simulink model "tia1_controller"  (R2023b)
settings: Solver=VariableStepAuto  StartTime=0  StopTime=20e-4  RelTol=1e-3
values from neighbouring files (symbols this model uses):
  fNoiseSampling = 1 / (rpFloor(2,1) - rpFloor(1,1))    [Laser_n_PID_initializer.m]
  fsampling = 125e6    (= 125000000)    [Laser_n_PID_initializer.m]
  initialWaitTime = 8e-4    (= 0.0008)    [Laser_n_PID_initializer.m]
  nDelay = ceil(350*.5)    [Laser_n_PID_initializer.m]    (also in bode_check_stability_w_time_delay.m = 319)
  s = estimate_iir_transfer_function(x,y,3,1)    [linearModelization.m]
libraries: slctrl_linear x4, spsFirstOrderFilterLib x3, slpidlib x1
settings Model: Creator=lastline  LastModifiedBy=lastline

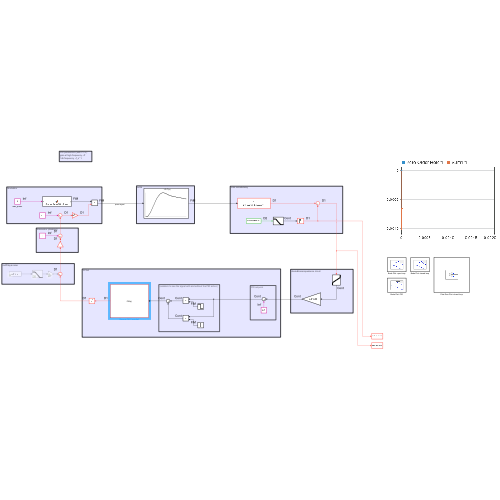
[thumbnail: Simulink's stored preview of the top-level diagram]
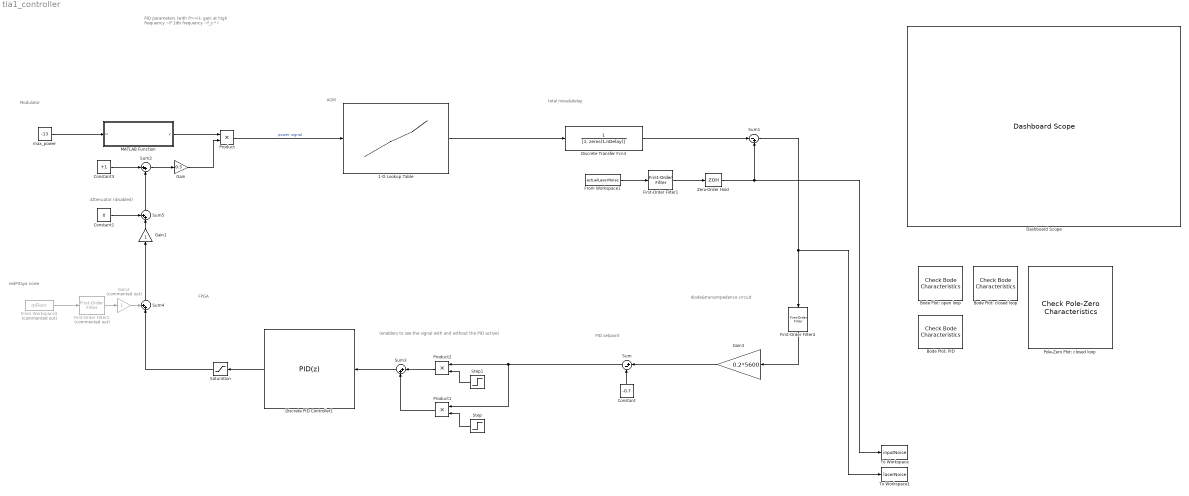
== system tia1_controller ==
  note: PID parameters (with P>>I):
      | gain at high frequency ~P
      | 1db frequency ~f_s * I
  note: PID setpoint
  note: (enablers to see the signal with and without the PID active)
  note: FPGA
  note: diode&transimpedance circuit
  note: Attenuator (disabled)
  note: AOM
  note: Modulator
  note: total noise&delay
  note: redPitaya noise
  1-D Lookup Table : Lookup_n-D  NumberOfTableDimensions=1  BreakpointsForDimension1=linspace(0, 1.58e-4, 250)  Table=0.7/0.0165796/(5600*0.2)*[0.00094876, 0.00102912, 0.00104173, 0.00106448, 0.00103857, 0.00100141, 0.00101933, 0.00100616, 0.00097746, 0.00121732, 0.00134761, 0.00150802, 0.00188835, 0.0021115 , 0.00246877, 0.00279502, 0.00315454, 0.0035255 , 0.00394097, 0.00436382, 0.00480437, 0.00527323, 0.00575644, 0.00627402, 0.00681823, 0.00736118, 0.00793556, 0.00852683, 0.00913098, 0.00972158, 0.01035586, 0.01102776, 0.0116796 , 0.01234212, 0.01306885, 0.0137567 , 0.01445381, 0.0151505 , 0.01585035, 0.01657956, 0.01728462, 0.01802811, 0.01875558, 0.01950813, 0.02025514, 0.02102895, 0.02180866, 0.02259664, 0.0233524 , 0.02406897, 0.02477072, 0.02553684, 0.02631157, 0.02703981, 0.02778477, 0.02851065, 0.02925919, 0.02997621, 0.03066793, 0.03135128, 0.0320296 , 0.03274458, 0.03341281, 0.03413072, 0.03476723, 0.0354006 , 0.03607709, 0.03668184, 0.03729911, 0.0378791 , 0.03846521, 0.0390453 , 0.03960121, 0.04011368, 0.04065807, 0.04118766, 0.04169539, 0.04217082, 0.0426283 , 0.04311696, 0.0435708 , 0.0439849 , 0.04437042, 0.04474889, 0.04514842, 0.04550796, 0.04586307, 0.04611688, 0.04647122, 0.04671718, 0.04707288, 0.04724069, 0.04745658, 0.04780167, 0.0479343 , 0.04808488, 0.04829364, 0.04849163, 0.04860279, 0.04865673, 0.04874706, 0.04886116, 0.04897224, 0.04908539, 0.04914333, 0.04916859, 0.04918415, 0.04919929, 0.04919949, 0.04918844, 0.0491581 , 0.04909332, 0.04902933, 0.04893137, 0.04879004, 0.04870624, 0.04865411, 0.04858254, 0.04848512, 0.04832172, 0.04815615, 0.04800017, 0.04790875, 0.04778889, 0.04761694, 0.04742341, 0.04726704, 0.04718501, 0.04700808, 0.04677664, 0.04662498, 0.04650092, 0.04634307, 0.04607253, 0.04590273, 0.04581645, 0.04568616, 0.04540447, 0.04523153, 0.0451333 , 0.04501928, 0.04482289, 0.04460957, 0.0444905 , 0.0444136 , 0.04426863, 0.04405665, 0.0439024 , 0.04381264, 0.04372158, 0.0436426 , 0.04347625, 0.04336099, 0.04321188, 0.04310523, 0.04304013, 0.04297429, 0.04289107, 0.04273544, 0.04258686, 0.0424759 , 0.04239794, 0.04236981, 0.04229522, 0.04221052, 0.04209073, 0.04197017, 0.04189005, 0.04178447, 0.04168274, 0.04166642, 0.04162506, 0.04155631, 0.04144807, 0.04133527, 0.04127493, 0.04118388, 0.04109912, 0.04101747, 0.04099294, 0.04096444, 0.04093825, 0.04089439, 0.04081889, 0.04076137, 0.04072337, 0.04064599, 0.0405364 , 0.04043972, 0.04039083, 0.04034431, 0.04030449, 0.04026617, 0.04022117, 0.04017923, 0.04012702, 0.04004417, 0.03997472, 0.03988416, 0.03978438, 0.03975578, 0.03968915, 0.03963203, 0.03959104, 0.03955679, 0.03953011, 0.03948652, 0.0394475 , 0.0393199 , 0.03924009, 0.03918222, 0.03910691, 0.03903237, 0.03894742, 0.03890655, 0.03889474, 0.03884979, 0.03882239, 0.03875444, 0.03868378, 0.03863993, 0.03856258, 0.03846697, 0.03834077, 0.03827951, 0.03826207, 0.03821381, 0.03818688, 0.03812229, 0.03809234, 0.03805151, 0.03796007, 0.03787821, 0.03773854, 0.03766482, 0.03762769, 0.03755333, 0.03751379, 0.03747958, 0.03744132, 0.03740655, 0.03731694, 0.0372496 , 0.03713154, 0.03703423, 0.03696138, 0.0368748 , 0.03684136, 0.03680855, 0.03677881]  InternalRulePriority=Speed  RndMeth=Simplest
  Bode Plot: PID : slctrl_linear/Check Bode  Characteristics  InstantiateOnLoad=on  SaveOperatingPoints=off  LinearizationIOs={'/Gain3', 1, 'in', 'off', '';'/Saturation', 1, 'out', 'on', ''}  LinearizeAt=SnapshotTimes  SnapshotTimes=[0]  TriggerType=rising  SampleTime=auto  RateConversionMethod=zoh  PreWarpFreq=10  UseExactDelayModel=off  UseFullBlockNameLabels=off  UseBusSignalLabels=on  enabled=on  stopWhenAssertionFail=off  export=off  ViewDlgPos=[1936 106 510 390]  OpenViewOnLoad=on  LaunchViewOnOpen=on  FrequencyUnits=rad/s  MagnitudeUnits=dB  PhaseUnits=deg  TimeUnits=seconds  EnableUpperBound=off  UpperBoundFrequencies=[]  UpperBoundMagnitudes=[]  EnableLowerBound=off  LowerBoundFrequencies=[]  LowerBoundMagnitudes=[]
      settings: LibrarySourceBlock=slctrlblks/Linear Analysis Plots/Bode Plot  SaveToWorkspace=off  SaveName=sys
  Bode Plot: closed loop : slctrl_linear/Check Bode  Characteristics  InstantiateOnLoad=on  SaveOperatingPoints=off  LinearizationIOs={'/Zero-Order Hold', 1, 'in', 'off', '';'/Sum1', 1, 'out', 'off', ''}  LinearizeAt=SnapshotTimes  SnapshotTimes=[0]  TriggerType=rising  SampleTime=auto  RateConversionMethod=zoh  PreWarpFreq=10  UseExactDelayModel=off  UseFullBlockNameLabels=off  UseBusSignalLabels=on  enabled=on  stopWhenAssertionFail=off  export=off  ViewDlgPos=[2464 597 510 390]  OpenViewOnLoad=off  LaunchViewOnOpen=on  FrequencyUnits=rad/s  MagnitudeUnits=dB  PhaseUnits=deg  TimeUnits=seconds  EnableUpperBound=off  UpperBoundFrequencies=[]  UpperBoundMagnitudes=[]  EnableLowerBound=off  LowerBoundFrequencies=[]  LowerBoundMagnitudes=[]
      settings: LibrarySourceBlock=slctrlblks/Linear Analysis Plots/Bode Plot  SaveToWorkspace=off  SaveName=sys
  Bode Plot: open loop : slctrl_linear/Check Bode  Characteristics  InstantiateOnLoad=on  SaveOperatingPoints=off  LinearizationIOs={'/Sum1', 1, 'in', 'off', '';'/Discrete Transfer Fcn3', 1, 'out', 'on', ''}  LinearizeAt=SnapshotTimes  SnapshotTimes=[0]  TriggerType=rising  SampleTime=auto  RateConversionMethod=zoh  PreWarpFreq=10  UseExactDelayModel=off  UseFullBlockNameLabels=off  UseBusSignalLabels=on  enabled=on  stopWhenAssertionFail=off  export=off  ViewDlgPos=[1936 598 510 390]  OpenViewOnLoad=on  LaunchViewOnOpen=on  FrequencyUnits=rad/s  MagnitudeUnits=dB  PhaseUnits=deg  TimeUnits=seconds  EnableUpperBound=off  UpperBoundFrequencies=[]  UpperBoundMagnitudes=[]  EnableLowerBound=off  LowerBoundFrequencies=[]  LowerBoundMagnitudes=[]
      settings: LibrarySourceBlock=slctrlblks/Linear Analysis Plots/Bode Plot  SaveToWorkspace=off  SaveName=sys
  Constant : Constant  Value=-0.7
  Constant1 : Constant  Value=0
  Constant3 : Constant  Value=+1
  Dashboard Scope : DashboardScope
  Discrete Transfer Fcn3 : DiscreteTransferFcn  Denominator=[1, zeros(1,nDelay)]  a0EqualsOne=on
  Discrete PID Controller1 : slpidlib/PID Controller  Controller=PID  Form=Parallel  TimeDomain=Discrete-time  UseExternalTs=off  SampleTime=1/fsampling  IntegratorMethod=Forward Euler  FilterMethod=Forward Euler  ControllerParametersSource=internal  P=1/2  I=0.03/2  UseKiTs=on  D=0  N=100  UseFilter=off  TunerSelectOption=Transfer Function Based (PID Tuner App)  InitialConditionSource=internal  InitialConditionForIntegrator=0  InitialConditionForFilter=0  DifferentiatorICPrevScaledInput=0  ExternalReset=none  TrackingMode=off  Kt=1  LimitOutput=off  SatLimitsSource=internal  UpperSaturationLimit=1  LowerSaturationLimit=-1  LinearizeAsGain=off  AntiWindupMode=clamping  Kb=1  LimitIntegrator=off  UpperIntegratorSaturationLimit=1  LowerIntegratorSaturationLimit=-1  POutMin=[]  POutMax=[]  IOutMin=[]  IOutMax=[]  DOutMin=[]  DOutMax=[]  NOutMin=[]  NOutMax=[]  SumOutMin=[]  SumOutMax=[]  SaturationOutMin=[]  SaturationOutMax=[]  PParamMin=[]  PParamMax=[]  IParamMin=[]  IParamMax=[]  DParamMin=[]  DParamMax=[]  NParamMin=[]  NParamMax=[]  KbParamMin=[]  KbParamMax=[]  KtParamMin=[]  KtParamMax=[]  KbOutMin=[]  KbOutMax=[]  KtOutMin=[]  KtOutMax=[]  IntegratorOutMin=[]  IntegratorOutMax=[]  FilterOutMin=[]  FilterOutMax=[]  SumI1OutMin=[]  SumI1OutMax=[]  SumI2OutMin=[]  SumI2OutMax=[]  SumI3OutMin=[]  SumI3OutMax=[]  SumI4OutMin=[]  SumI4OutMax=[]  SumDOutMin=[]  SumDOutMax=[]  DifferentiatorOutMin=[]  DifferentiatorOutMax=[]  FilterDiffOutCoefMin=[]  FilterDiffOutCoefMax=[]  ReciprocalOutMin=[]  ReciprocalOutMax=[]  SumDenOutMin=[]  SumDenOutMax=[]  SumNumOutMin=[]  SumNumOutMax=[]  DivideOutMin=[]  DivideOutMax=[]  UdiffTsProdOutMin=[]  UdiffTsProdOutMax=[]  NTsProdOutMin=[]  NTsProdOutMax=[]  UintegralTsProdOutMin=[]  UintegralTsProdOutMax=[]  UngainTsProdOutMin=[]  UngainTsProdOutMax=[]  ClampingZeroOutDataTypeStr=Inherit: Inherit via back propagation  ClampingZeroOutMin=[]  ClampingZeroOutMax=[]  FilterDenConstantOutDataTypeStr=Inherit: Inherit via back propagation  FilterDenConstantOutMin=[]  FilterDenConstantOutMax=[]  PCopyOutDataTypeStr=Inherit: Inherit via back propagation  PCopyOutMin=[]  PCopyOutMax=[]  NCopyOutDataTypeStr=Inherit: Inherit via back propagation  NCopyOutMin=[]  NCopyOutMax=[]  IntegratorContinuousStateAttributes=''  IntegratorStateMustResolveToSignalObject=off  IntegratorRTWStateStorageClass=Auto  FilterContinuousStateAttributes=''  FilterStateMustResolveToSignalObject=off  FilterRTWStateStorageClass=Auto  ParallelPVariant=InternalParameters  IdealPVariant=Disabled  IVariant=InternalParameters  DVariant=InternalParameters  IntegratorVariant=Discrete  SatVariant=Disabled  AWVariant=Passthrough  PCopyVariant=Disabled  TRVariant=Disabled  FdbkBlocksVariant=Forward  IdealPFdbkVariant=Disabled  SatFdbkVariant=Disabled  DerivativeFilterVariant=Differentiator  NVariant=Passthrough  NCopyVariant=Disabled_SignalSpec  FilterICVariant=InternalICsDifferentiator  IntegratorICVariant=InternalICs  ExternalResetVariant=Disabled  TRSumVariant=Passthrough  SumFdbkVariant=Disabled  SumVariant=Sum_PID  TsampFilterVariant=InternalTs  TsampNgainVariant=Passthrough  TsampIntegralVariant=Disabled_SignalSpec  ExternalSaturationOutDataTypeStr=Inherit: Same as second input
      settings: LibrarySourceBlock=simulink/Discrete/Discrete PID Controller
  First-Order Filter1 : spsFirstOrderFilterLib/First-Order Filter  FilterType=Lowpass  Tc=1/200e3  Ts=0  Initialize=on  Vac_Init=[0, 0, 60]  Vdc_Init=0  PlotResponse=off  FreqRange="[0,  200,  1]"
  First-Order Filter2 : spsFirstOrderFilterLib/First-Order Filter  Commented=on  FilterType=Lowpass  Tc=1/(200e3*2*pi)  Ts=0  Initialize=on  Vac_Init=[0, 0, 60]  Vdc_Init=0  PlotResponse=off  FreqRange="[0,  200,  1]"
  First-Order Filter4 : spsFirstOrderFilterLib/First-Order Filter  FilterType=Lowpass  Tc=(10e-12*5600)  Ts=0  Initialize=on  Vac_Init=[0, 0, 60]  Vdc_Init=0  PlotResponse=off  FreqRange="[0,  200,  1]"
  From Workspace1 : FromWorkspace  VariableName=actualLaserNoise  SampleTime=1/fNoiseSampling  OutputAfterFinalValue=Setting to zero
  From Workspace3 : FromWorkspace  Commented=on  VariableName=rpFloor  SampleTime=1/fNoiseSampling  OutputAfterFinalValue=Setting to zero
  Gain : Gain  Gain=0.5
  Gain1 : Gain
  Gain2 : Gain  Commented=on
  Gain3 : Gain  Gain=0.2*5600
  MATLAB Function : MATLAB Function  TreatAsAtomicUnit=on
  Pole-Zero Plot: closed loop : slctrl_linear/Check Pole-Zero Characteristics  InstantiateOnLoad=on  SaveOperatingPoints=off  LinearizationIOs={'/Zero-Order Hold', 1, 'in', 'off', '';'/Sum1', 1, 'out', 'off', ''}  LinearizeAt=SnapshotTimes  SnapshotTimes=[0]  TriggerType=rising  SampleTime=auto  RateConversionMethod=zoh  PreWarpFreq=10  UseExactDelayModel=off  UseFullBlockNameLabels=off  UseBusSignalLabels=off  enabled=on  stopWhenAssertionFail=off  export=off  ViewDlgPos=[2986 110 845 873]  LaunchViewOnOpen=on  OpenViewOnLoad=on  FrequencyUnits=rad/s  MagnitudeUnits=dB  PhaseUnits=deg  TimeUnits=seconds  EnableSettlingTime=off  SettlingTime=[]  EnablePercentOvershoot=off  PercentOvershoot=[]  EnableDampingRatio=off  DampingRatio=[]  EnableNaturalFrequency=off  NaturalFrequencyBound=>=  NaturalFrequency=[]
      settings: LibrarySourceBlock=slctrlblks/Linear Analysis Plots/Pole-Zero Plot  SaveToWorkspace=off  SaveName=sys
  Product : Product
  Product1 : Product
  Product2 : Product
  Saturation : Saturate  UpperLimit=1  LowerLimit=-1
  Step : Step  Time=initialWaitTime  SampleTime=0
  Step1 : Step  Time=1/fsampling  Before=1  After=0  SampleTime=0
  Sum : Sum  Inputs=|+-
  Sum1 : Sum  Inputs=|-+
  Sum2 : Sum  Inputs=|++
  Sum3 : Sum  Inputs=|++
  Sum4 : Sum  Inputs=++|
  Sum5 : Sum  Inputs=++|
  To Workspace : ToWorkspace  VariableName=inputNoise  SaveFormat=Structure With Time  SampleTime=-1
  To Workspace1 : ToWorkspace  VariableName=laserNoise  SaveFormat=Timeseries  SampleTime=-1
  Zero-Order Hold : ZeroOrderHold  SampleTime=1/fsampling
  max_power : Constant  Value=-13
  wires:
  Product/1 -> 1-D Lookup Table/1  "power signal"
  max_power/1 -> MATLAB Function/1(u)
  MATLAB Function/1(y) -> Product/1
  Gain/1 -> Product/2
  Sum2/1 -> Gain/1
  Constant3/1 -> Sum2/1
  From Workspace3/1 -> First-Order Filter2/1
  Sum4/1 -> Gain1/1
  First-Order Filter2/1 -> Gain2/1
  Discrete PID Controller1/1 -> Saturation/1
  Gain1/1 -> Sum5/2
  Sum5/1 -> Sum2/2
  Constant1/1 -> Sum5/1
  Saturation/1 -> Sum4/2
  Gain2/1 -> Sum4/1
  Step/1 -> Product1/2
  From Workspace1/1 -> First-Order Filter1/1
  Product2/1 -> Sum3/1
  Step1/1 -> Product2/2
  Product1/1 -> Sum3/2
  First-Order Filter1/1 -> Zero-Order Hold/1
  Sum3/1 -> Discrete PID Controller1/1
  Zero-Order Hold/1 -> Sum1/2, To Workspace/1
  Sum1/1 -> To Workspace1/1, First-Order Filter4/1
  Discrete Transfer Fcn3/1 -> Sum1/1
  1-D Lookup Table/1 -> Discrete Transfer Fcn3/1
  Sum/1 -> Product2/1, Product1/1
  Gain3/1 -> Sum/1
  Constant/1 -> Sum/2
  First-Order Filter4/1 -> Gain3/1

== matlab function tia1_controller/MATLAB Function ==
  data: u input; y output
function y = dBm_to_PiezoDrivingPower(u)

y = 10 ^ (u / 10 - 3);
